simulink model "dc_dc_fb_fszvs"  (Simulink 7.9)
settings: Solver=ode23tb  StartTime=0.0  StopTime=0.001  MaxStep=2e-7  RelTol=1e-3  AbsTol=.01
libraries: powerlib x19
settings Model: Creator=lanyi  LastModifiedBy=lanyi
settings OptimizationCC: InlineInvariantSignals=on  InitFltsAndDblsToZero=on
settings DebuggingCC: SaveWithParameterizedLinksMsg=none  SignalResolutionControl=TryResolveAllWithWarning  MultiTaskDSMMsg=warning  MultiTaskCondExecSysMsg=none  FcnCallInpInsideContextMsg=Use local settings  StrictBusMsg=None
settings RTWCC: IncludeERTFirstTime=on
settings GRTTargetCC: TargetFcnLib=ansi_tfl_tmw.mat  CombineOutputUpdateFcns=off  GRTInterface=on

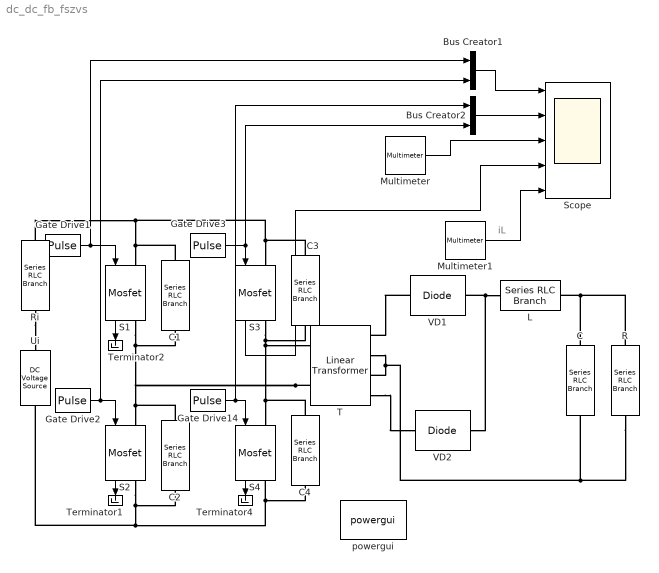
== system dc_dc_fb_fszvs ==
  note: iL
  Bus Creator1 : BusCreator  DialogController=Simulink.DDGSource_Bus  Inputs=2
  Bus Creator2 : BusCreator  DialogController=Simulink.DDGSource_Bus  Inputs=2
  C : powerlib/Elements/Series RLC Branch  LConnTagsString=__new0  RConnTagsString=__new0  BranchType=RLC  Resistance=0  Inductance=0  SetiL0=off  InitialCurrent=0  Capacitance=1e-4  Setx0=off  InitialVoltage=0  Measurements=None
  C{1..4} (4 alike) : powerlib/Elements/Series RLC Branch  LConnTagsString=__new0  RConnTagsString=__new0  BranchType=RLC  Resistance=0  Inductance=0  SetiL0=off  InitialCurrent=0  Capacitance=1e-7  Setx0=off  InitialVoltage=0  Measurements=None
  Gate Drive1 : DiscretePulseGenerator  PulseType=Time based  Period=50e-6  PulseWidth=47
  Gate Drive14 : DiscretePulseGenerator  PulseType=Time based  Period=50e-6  PulseWidth=47  PhaseDelay=5e-6
  Gate Drive2 : DiscretePulseGenerator  PulseType=Time based  Period=50e-6  PulseWidth=47  PhaseDelay=25e-6
  Gate Drive3 : DiscretePulseGenerator  PulseType=Time based  Period=50e-6  PulseWidth=47  PhaseDelay=30e-6
  L : powerlib/Elements/Series RLC Branch  LConnTagsString=__new0  RConnTagsString=__new0  BranchType=RLC  Resistance=0  Inductance=5e-5  SetiL0=off  InitialCurrent=0  Capacitance=inf  Setx0=off  InitialVoltage=0  Measurements=Branch voltage and current
  Multimeter : powerlib/Measurements/Multimeter  PhasorSimulation=off  OutputType=Complex  sel=[3 7]  L=10  Gain=[1 1]  yselected={'Uw1: T','Iw1: T'};  PSBOutputType=1  PSBequivalent=0  AxesSetting=[0,0.1,-100,100]  Display=0  SavedBlockNames=-11
  Multimeter1 : powerlib/Measurements/Multimeter  PhasorSimulation=off  OutputType=Complex  sel=6  L=10  Gain=1  yselected={'Ib: L'};  PSBOutputType=1  PSBequivalent=0  AxesSetting=[0,0.1,-100,100]  Display=0  SavedBlockNames=-11
  R : powerlib/Elements/Series RLC Branch  LConnTagsString=__new0  RConnTagsString=__new0  BranchType=RLC  Resistance=0.4  Inductance=0  SetiL0=off  InitialCurrent=0  Capacitance=inf  Setx0=off  InitialVoltage=0  Measurements=Branch voltage
  Ri : powerlib/Elements/Series RLC Branch  LConnTagsString=__new0  RConnTagsString=__new0  BranchType=RLC  Resistance=.01  Inductance=0  SetiL0=off  InitialCurrent=0  Capacitance=inf  Setx0=off  InitialVoltage=0  Measurements=None
  S{1..4} (4 alike) : powerlib/Power Electronics/Mosfet  Ron=0.05  Lon=1e-9  Rd=0.05  Vfd=0  IC=0  Rs=100  Cs=1e-8  Measurements=on
  Scope : Scope  NumInputPorts=5
      settings: TimeRange=0.0001  YMin=-0.5~-0.5~-100~-20~0  YMax=1.5~1.5~100~60~40  SampleTime=1e-7
  T : powerlib/Elements/Linear Transformer  LConnTagsString=a|b  RConnTagsString=A|B|C|D  UNITS=pu  NominalPower=[500 20000 ]  winding1="[ 100  0.002  0.02 ]"  winding2="[ 50  0.002  0.02 ]"  ThreeWindings=on  winding3=[ 50 0.002 0.02 ]  RmLm=[ 500 20 ]  Measurements=All voltages and currents  DataType=off
  Terminator1 : Terminator
  Terminator2 : Terminator
  Terminator4 : Terminator
  Ui : powerlib/Electrical Sources/DC Voltage Source  Amplitude=50  Measurements=None
  VD1 : powerlib/Power Electronics/Diode  Ron=0.01  Lon=0  Vf=0.8  IC=0  UseSnubber=off  Rs=100  Cs=1e-9  Measurements=off
  VD2 : powerlib/Power Electronics/Diode  Ron=0.01  Lon=0  Vf=0.8  IC=0  UseSnubber=off  Rs=100  Cs=1e-9  Measurements=off
  powergui : powerlib/powergui  Priority=1  SimulationMode=Continuous  SolverType=Tustin  SampleTime=50e-6  frequency=60  SPID=off  DisableSnubberDevices=off  DisableRonSwitches=off  DisableVfSwitches=off  SwTol=0  Interpol=off  DisplayEquations=off  FunctionMessages=off  frequencyindice=60  Pbase=100e6  ErrMax=1e-4  Iterations=50  UnitsV=kV  UnitsW=MW  echomessages=off  HookPort=off  EnableUseOfTLC=off  x0status=blocks  RestoreLinks=warning  ResistiveCurrentMeasurement=off  Ylog=off  Xlog=on  ShowGrid=off  save=off  variable=ZData  ZoomFFT=off  StartTime=0.0  cycles=1  DisplayStyle=1  FreqAxis=off  MaxFrequency=1000  frequencyindicesteady=1  display=off  methode=off
  wires:
  Gate Drive1/1 -> S1/1, Bus Creator1/1
  Multimeter/1 -> Scope/3
  Gate Drive2/1 -> S2/1, Bus Creator1/2
  S1/1 -> Terminator2/1
  S2/1 -> Terminator1/1
  S4/1 -> Terminator4/1
  Gate Drive3/1 -> S3/1, Bus Creator2/2
  Gate Drive14/1 -> S4/1, Bus Creator2/1
  Bus Creator1/1 -> Scope/1
  Bus Creator2/1 -> Scope/2
  S3/1 -> Scope/4
  Multimeter1/1 -> Scope/5
  connections:
  Ui/LConn1 -- S2/RConn1 -- C2/LConn1 -- S4/RConn1 -- C4/LConn1
  S3/RConn1 -- T/LConn1 -- S4/LConn1 -- C4/RConn1 -- C3/LConn1
  Ri/RConn1 -- S3/LConn1 -- C3/RConn1 -- S1/LConn1 -- C1/RConn1
  T/LConn2 -- S1/RConn1 -- C1/LConn1 -- S2/LConn1 -- C2/RConn1
  VD1/LConn1 -- T/RConn1
  R/LConn1 -- L/RConn1 -- C/RConn1
  VD2/RConn1 -- VD1/RConn1 -- L/LConn1
  R/RConn1 -- T/RConn2 -- T/RConn3 -- C/LConn1
  T/RConn4 -- VD2/LConn1
  Ri/LConn1 -- Ui/RConn1
